simulink subsystem "bh_COMP_sys_Newton"  (R2022b)
settings: Solver=VariableStepAuto  StartTime=0.0  StopTime=10.0  RelTol=1e-3
undefined symbols (not defined in the file or in its folder): IC_T, params_T
libraries: simulink x1, simulink_extras x1
settings Model: Creator=bhorton  LastModifiedBy=bhorton
settings DebuggingCC: UnconnectedInputMsg=warning  UnconnectedOutputMsg=warning  UnconnectedLineMsg=warning
settings ModelReferenceCC: EnableRefExpFcnMdlSchedulingChecks=on
settings RTWCC: DLArmComputeVersion=19.05

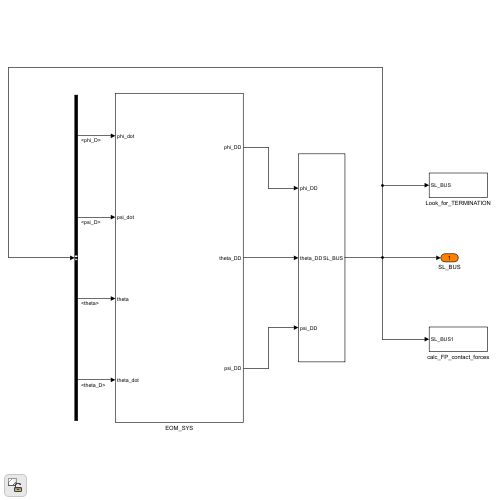
[thumbnail: Simulink's stored preview of the top-level diagram]
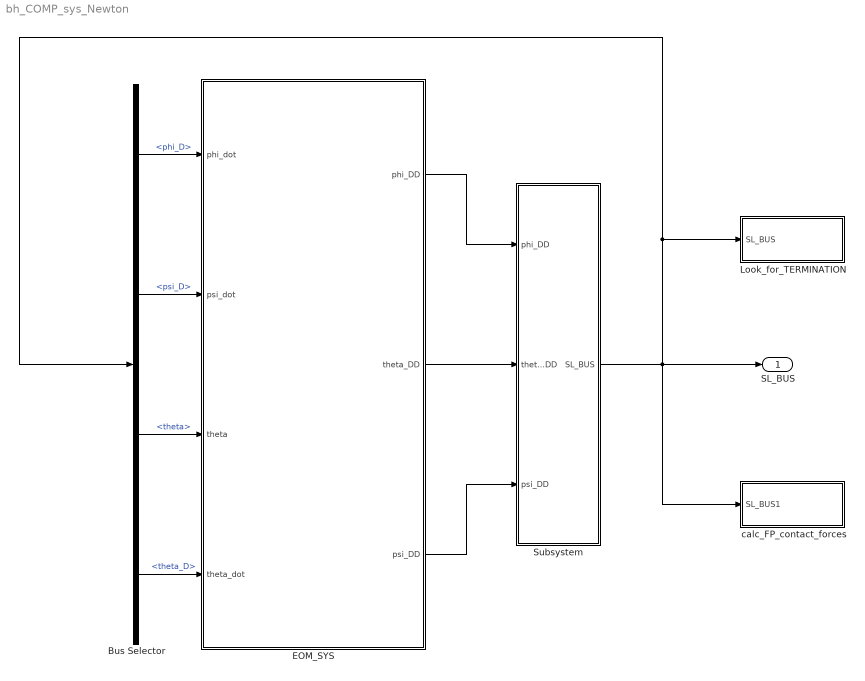
== system bh_COMP_sys_Newton ==
  Bus Selector : BusSelector  OutputSignals=phi_D,psi_D,theta,theta_D
  EOM_SYS : Subsystem
  Look_for_TERMINATION : Subsystem
  Subsystem : Subsystem
  calc_FP_contact_forces : Subsystem
  SL_BUS : Outport
  wires:
  EOM_SYS/3(psi_DD) -> Subsystem/3(psi_DD)
  EOM_SYS/2(theta_DD) -> Subsystem/2(theta_DD)
  EOM_SYS/1(phi_DD) -> Subsystem/1(phi_DD)
  Bus Selector/2 -> EOM_SYS/2(psi_dot)  "<psi_D>"
  Bus Selector/1 -> EOM_SYS/1(phi_dot)  "<phi_D>"
  Bus Selector/3 -> EOM_SYS/3(theta)  "<theta>"
  Bus Selector/4 -> EOM_SYS/4(theta_dot)  "<theta_D>"
  Subsystem/1(SL_BUS) -> SL_BUS/1, Look_for_TERMINATION/1(SL_BUS), Bus Selector/1, calc_FP_contact_forces/1(SL_BUS1)

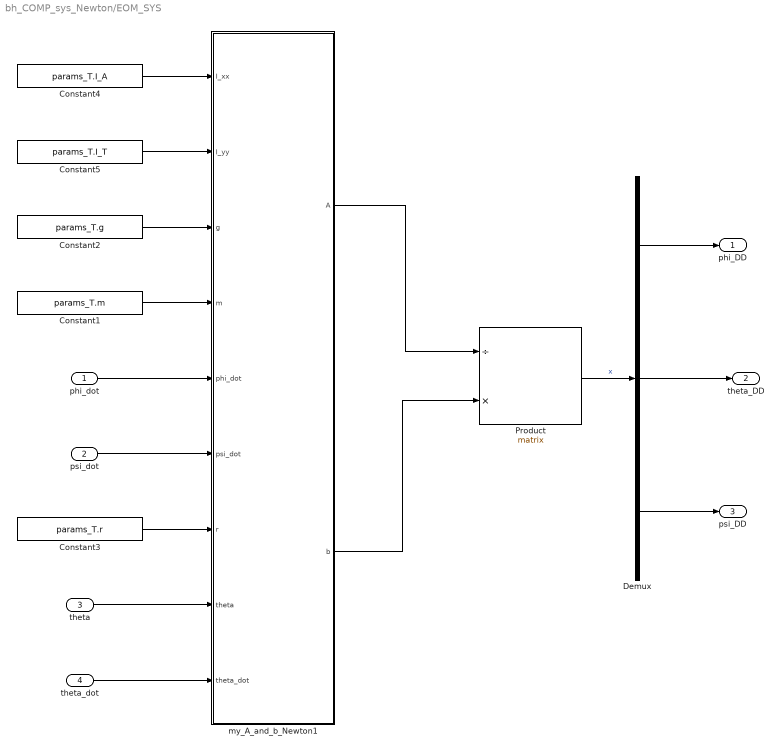
== system bh_COMP_sys_Newton/EOM_SYS ==
  phi_dot : Inport
  psi_dot : Inport  Port=2
  theta : Inport  Port=3
  theta_dot : Inport  Port=4
  Constant1 : Constant  Value=params_T.m
  Constant2 : Constant  Value=params_T.g
  Constant3 : Constant  Value=params_T.r
  Constant4 : Constant  Value=params_T.I_A
  Constant5 : Constant  Value=params_T.I_T
  Demux : Demux  Outputs=3
  Product : Product  Inputs=/*  Multiplication=Matrix(*)
  my_A_and_b_Newton1 : MATLAB Function  TreatAsAtomicUnit=on
  phi_DD : Outport
  theta_DD : Outport  Port=2
  psi_DD : Outport  Port=3
  wires:
  Constant5/1 -> my_A_and_b_Newton1/2(I_yy)
  Constant4/1 -> my_A_and_b_Newton1/1(I_xx)
  Constant2/1 -> my_A_and_b_Newton1/3(g)
  Constant1/1 -> my_A_and_b_Newton1/4(m)
  theta/1 -> my_A_and_b_Newton1/8(theta)
  theta_dot/1 -> my_A_and_b_Newton1/9(theta_dot)
  psi_dot/1 -> my_A_and_b_Newton1/6(psi_dot)
  phi_dot/1 -> my_A_and_b_Newton1/5(phi_dot)
  Demux/3 -> psi_DD/1
  Demux/2 -> theta_DD/1
  Constant3/1 -> my_A_and_b_Newton1/7(r)
  my_A_and_b_Newton1/2(b) -> Product/2
  my_A_and_b_Newton1/1(A) -> Product/1
  Demux/1 -> phi_DD/1
  Product/1 -> Demux/1  "x"

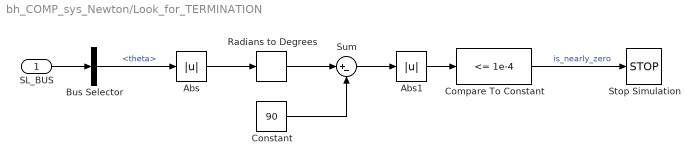
== system bh_COMP_sys_Newton/Look_for_TERMINATION ==
  SL_BUS : Inport
  Abs : Abs  SaturateOnIntegerOverflow=off
  Abs1 : Abs  SaturateOnIntegerOverflow=off
  Bus Selector : BusSelector  OutputSignals=theta
  Compare To Constant : simulink/Logic and Bit Operations/Compare To Constant  relop=<=  const=1e-4  OutDataTypeStr=boolean
  Constant : Constant  Value=90
  Radians to Degrees : simulink_extras/Transformations/Radians to Degrees
  Stop Simulation : Stop
  Sum : Sum  Inputs=|+-
  wires:
  Compare To Constant/1 -> Stop Simulation/1  "is_nearly_zero"
  Abs1/1 -> Compare To Constant/1
  Sum/1 -> Abs1/1
  Constant/1 -> Sum/2
  Radians to Degrees/1 -> Sum/1
  Abs/1 -> Radians to Degrees/1
  Bus Selector/1 -> Abs/1  "<theta>"
  SL_BUS/1 -> Bus Selector/1

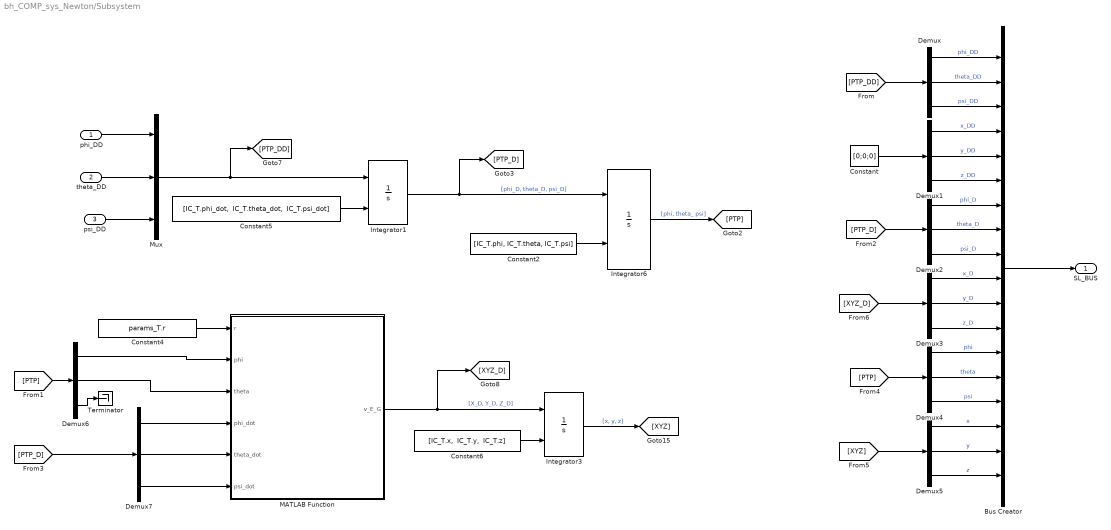
== system bh_COMP_sys_Newton/Subsystem ==
  phi_DD : Inport
  theta_DD : Inport  Port=2
  psi_DD : Inport  Port=3
  Bus Creator : BusCreator  Inputs=18
  Constant : Constant  Value=[0;0;0]
  Constant2 : Constant  Value="[IC_T.phi,  IC_T.theta,  IC_T.psi]"
  Constant4 : Constant  Value=params_T.r
  Constant5 : Constant  Value="[IC_T.phi_dot,  IC_T.theta_dot,  IC_T.psi_dot]"
  Constant6 : Constant  Value="[IC_T.x,  IC_T.y,  IC_T.z]"
  Demux{,1..7} (8 alike) : Demux  Outputs=3
  Integrator1 : Integrator  InitialConditionSource=external
  Integrator3 : Integrator  InitialConditionSource=external
  Integrator6 : Integrator  InitialConditionSource=external  WrapState=on  WrappedStateUpperValue=2*pi  WrappedStateLowerValue=0  AbsoluteTolerance=1e-8
  MATLAB Function : MATLAB Function  TreatAsAtomicUnit=on
  Mux : Mux  Inputs=3
  Terminator : Terminator
  SL_BUS : Outport
  wires:
  Integrator3/1 -> [XYZ]  "[x, y, z]"
  Constant6/1 -> Integrator3/2
  MATLAB Function/1(v_E_G) -> Integrator3/1, [XYZ_D]  "[X_D, Y_D, Z_D]"
  [PTP] -> Demux6/1
  Demux6/3 -> Terminator/1
  Demux6/2 -> MATLAB Function/3(theta)
  Demux6/1 -> MATLAB Function/2(phi)
  Demux7/3 -> MATLAB Function/6(psi_dot)
  Demux7/2 -> MATLAB Function/5(theta_dot)
  Demux7/1 -> MATLAB Function/4(phi_dot)
  [PTP_D] -> Demux7/1
  Constant4/1 -> MATLAB Function/1(r)
  [XYZ] -> Demux5/1
  [PTP] -> Demux4/1
  [XYZ_D] -> Demux3/1
  [PTP_D] -> Demux2/1
  Constant/1 -> Demux1/1
  [PTP_DD] -> Demux/1
  Demux4/3 -> Bus Creator/15  "psi"
  Demux5/1 -> Bus Creator/16  "x"
  Demux5/3 -> Bus Creator/18  "z"
  Demux4/1 -> Bus Creator/13  "phi"
  Demux4/2 -> Bus Creator/14  "theta"
  Demux5/2 -> Bus Creator/17  "y"
  Demux2/3 -> Bus Creator/9  "psi_D"
  Demux3/2 -> Bus Creator/11  "y_D"
  Demux3/1 -> Bus Creator/10  "x_D"
  Demux3/3 -> Bus Creator/12  "z_D"
  Demux2/1 -> Bus Creator/7  "phi_D"
  Demux2/2 -> Bus Creator/8  "theta_D"
  Demux1/3 -> Bus Creator/6  "z_DD"
  Demux1/2 -> Bus Creator/5  "y_DD"
  Demux1/1 -> Bus Creator/4  "x_DD"
  Demux/3 -> Bus Creator/3  "psi_DD"
  Demux/1 -> Bus Creator/1  "phi_DD"
  Demux/2 -> Bus Creator/2  "theta_DD"
  Bus Creator/1 -> SL_BUS/1
  Mux/1 -> Integrator1/1, [PTP_DD]
  phi_DD/1 -> Mux/1
  theta_DD/1 -> Mux/2
  psi_DD/1 -> Mux/3
  Constant5/1 -> Integrator1/2
  Constant2/1 -> Integrator6/2
  Integrator6/1 -> [PTP]  "[phi, theta_ psi]"
  Integrator1/1 -> [PTP_D], Integrator6/1  "[phi_D, theta_D, psi_D]"

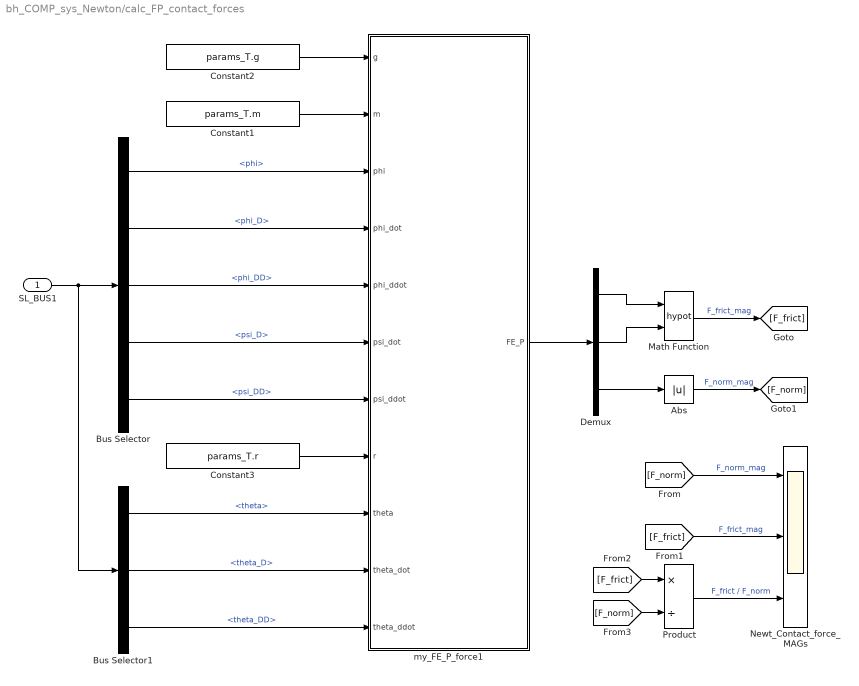
== system bh_COMP_sys_Newton/calc_FP_contact_forces ==
  SL_BUS1 : Inport
  Abs : Abs  SaturateOnIntegerOverflow=off
  Bus Selector : BusSelector  OutputSignals=phi,phi_D,phi_DD,psi_D,psi_DD
  Bus Selector1 : BusSelector  OutputSignals=theta,theta_D,theta_DD
  Constant1 : Constant  Value=params_T.m
  Constant2 : Constant  Value=params_T.g
  Constant3 : Constant  Value=params_T.r
  Demux : Demux  Outputs=3
  Math Function : Math  Operator=hypot
  Newt_Contact_force_MAGs : Scope  NumInputPorts=3
  Product : Product  Inputs=*/
  my_FE_P_force1 : MATLAB Function  TreatAsAtomicUnit=on
  wires:
  [F_norm] -> Product/2
  [F_frict] -> Product/1
  Product/1 -> Newt_Contact_force_MAGs/3  "F_frict / F_norm"
  Abs/1 -> [F_norm]  "F_norm_mag"
  Math Function/1 -> [F_frict]  "F_frict_mag"
  [F_frict] -> Newt_Contact_force_MAGs/2  "F_frict_mag"
  [F_norm] -> Newt_Contact_force_MAGs/1  "F_norm_mag"
  Demux/2 -> Math Function/2
  Demux/1 -> Math Function/1
  Demux/3 -> Abs/1
  my_FE_P_force1/1(FE_P) -> Demux/1
  Bus Selector1/3 -> my_FE_P_force1/11(theta_ddot)  "<theta_DD>"
  Bus Selector1/2 -> my_FE_P_force1/10(theta_dot)  "<theta_D>"
  Bus Selector1/1 -> my_FE_P_force1/9(theta)  "<theta>"
  Bus Selector/5 -> my_FE_P_force1/7(psi_ddot)  "<psi_DD>"
  Bus Selector/4 -> my_FE_P_force1/6(psi_dot)  "<psi_D>"
  Bus Selector/3 -> my_FE_P_force1/5(phi_ddot)  "<phi_DD>"
  Bus Selector/2 -> my_FE_P_force1/4(phi_dot)  "<phi_D>"
  Bus Selector/1 -> my_FE_P_force1/3(phi)  "<phi>"
  Constant3/1 -> my_FE_P_force1/8(r)
  Constant2/1 -> my_FE_P_force1/1(g)
  Constant1/1 -> my_FE_P_force1/2(m)
  SL_BUS1/1 -> Bus Selector/1, Bus Selector1/1

== matlab function bh_COMP_sys_Newton/calc_FP_contact_forces/my_FE_P_force1 ==
  data: g input; FE_P output; m input; phi input; phi_dot input; phi_ddot input; psi_dot input; psi_ddot input; r input; theta input; theta_dot input; theta_ddot input
function FE_P = my_FE_P_force(g,m,phi,phi_dot,phi_ddot,psi_dot,psi_ddot,r,theta,theta_dot,theta_ddot)
%#codegen

%    This function was generated by the Symbolic Math Toolbox version 9.2.
%    27-Oct-2022 13:27:01

FE_P = [-m.*r.*(-psi_ddot.*sin(phi)-phi_dot.*psi_dot.*cos(phi)-theta_ddot.*cos(phi).*cos(theta)+phi_ddot.*sin(phi).*sin(theta)+phi_dot.^2.*cos(phi).*sin(theta)+theta_dot.^2.*cos(phi).*sin(theta)+phi_dot.*theta_dot.*cos(theta).*sin(phi).*2.0);m.*r.*(-psi_ddot.*cos(phi)+phi_dot.*psi_dot.*sin(phi)+phi_ddot.*cos(phi).*sin(theta)+theta_ddot.*cos(theta).*sin(phi)-phi_dot.^2.*sin(phi).*sin(theta)-theta_dot.^2.*sin(phi).*sin(theta)+phi_dot.*theta_dot.*cos(phi).*cos(theta).*2.0);-m.*(-g+r.*theta_ddot.*sin(theta)+r.*theta_dot.^2.*cos(theta))];

== matlab function bh_COMP_sys_Newton/EOM_SYS/my_A_and_b_Newton1 ==
  data: I_xx input; A output; I_yy input; g input; m input; phi_dot input; psi_dot input; r input; theta input; theta_dot input; b output
function [A,b] = my_A_and_b_Newton(I_xx,I_yy,g,m,phi_dot,psi_dot,r,theta,theta_dot)
%#codegen

%    This function was generated by the Symbolic Math Toolbox version 9.2.
%    27-Oct-2022 13:27:01

A = reshape([I_xx.*sin(theta)+m.*r.^2.*sin(theta),0.0,I_yy.*cos(theta),0.0,-I_yy-m.*r.^2,0.0,-I_xx-m.*r.^2,0.0,0.0],[3,3]);
if nargout > 1
    b = [-I_xx.*phi_dot.*theta_dot.*cos(theta)-m.*phi_dot.*r.^2.*theta_dot.*cos(theta).*2.0;-m.*r.*(g.*sin(theta)+phi_dot.^2.*r.*cos(theta).*sin(theta)-phi_dot.*psi_dot.*r.*cos(theta))+I_yy.*phi_dot.^2.*cos(theta).*sin(theta)+I_xx.*phi_dot.*cos(theta).*(psi_dot-phi_dot.*sin(theta));I_xx.*theta_dot.*(psi_dot-phi_dot.*sin(theta))+I_yy.*phi_dot.*theta_dot.*sin(theta).*2.0];
end

== matlab function bh_COMP_sys_Newton/Subsystem/MATLAB Function ==
  data: r input; v_E_G output; phi input; theta input; phi_dot input; theta_dot input; psi_dot input
function v_E_G = LOC_calc_XYZ_G_vel(r, phi, theta, phi_dot, theta_dot, psi_dot)

v_E_G = ...
    [  r*(psi_dot*sin(phi) + theta_dot*cos(phi)*cos(theta) - phi_dot*sin(phi)*sin(theta));
       r*(phi_dot*cos(phi)*sin(theta) - psi_dot*cos(phi) + theta_dot*cos(theta)*sin(phi));
      -r*theta_dot*sin(theta) ];


end
